simulink library "IO"  (R2025a)
(part 5 of 6)

  raptor_can_rxmsg61 : Raptor_lib/CAN/raptor_can_rxmsg  canDefinition=struct('dbcFile', 'SR26_CAN2.dbc','message', 'BMS_553','comment', '','signals', {{'BMS_counterMsg553','BMS_module5Cell7Volt','BMS_module5Cell8Volt','BMS_module5Cell9Volt'}},'enabled', [ 1 1 1 1;],'scaled', [ 1 1 1 1;],'canBus', '''CAN2''','messageID', [ 553;],'idMask', [ 536870911;],'payloadMask', [],'payloadValue', [],'period', [ 0;],'mailbox', '''''','queueSize', [ 1;],'label', [ 0;],'ver', [ 2;],'showID', [ 0;],'showRaw', [ 0;],'showRawMsg', [ 0;],'useStartVals', [ 0;],'extendedId', [ 0;],'showAge', [ 1;],'useSimFunc', [ 0;],'sim_func_name', '''''','fill', [ 0;],'editID', [ 0;],'signalOrder', [ 2;],'signalAscDes', [ 2;],'msgLength', [ 8;])  canBus='CAN2'  mailbox=''  payloadMask=[]  payloadValue=[]  idMask=hex2dec('1FFFFFFF')  queueSize=1  showID=0  label=0  fill=0  id=553  showRaw=0  showAge=1  signalOrder=2  signalInfo={{struct('Name', 'BMS_module5Cell9Volt','StartBit', [ 48;],'SignalSize', [ 16;],'ByteOrder', 'LittleEndian','ValueType', 'SIGNED','Class', 'int16','Signed', [ 1;],'Factor', [ 0.001;],'Offset', [ 0;],'Min', [ -32.768;],'Max', [ 32.767;],'Units', 'V','StartVal', [ 0;],'Comment', 'Module 5 Cell 9 Voltage','Multiplexed', [ 0;],'Multiplexor', [ 0;],'MultiplexMode_Min', [],'MultiplexMode_Max', []),struct('Name', 'BMS_module5Cell8Volt','StartBit', [ 32;],'SignalSize', [ 16;],'ByteOrder', 'LittleEndian','ValueType', 'SIGNED','Class', 'int16','Signed', [ 1;],'Factor', [ 0.001;],'Offset', [ 0;],'Min', [ -32.768;],'Max', [ 32.767;],'Units', 'V','StartVal', [ 0;],'Comment', 'Module 5 Cell 8 Voltage','Multiplexed', [ 0;],'Multiplexor', [ 0;],'MultiplexMode_Min', [],'MultiplexMode_Max', []),struct('Name', 'BMS_module5Cell7Volt','StartBit', [ 16;],'SignalSize', [ 16;],'ByteOrder', 'LittleEndian','ValueType', 'SIGNED','Class', 'int16','Signed', [ 1;],'Factor', [ 0.001;],'Offset', [ 0;],'Min', [ -32.768;],'Max', [ 32.767;],'Units', 'V','StartVal', [ 0;],'Comment', 'Module 5 Cell 7 Voltage','Multiplexed', [ 0;],'Multiplexor', [ 0;],'MultiplexMode_Min', [],'MultiplexMode_Max', []),struct('Name', 'BMS_counterMsg553','StartBit', [ 0;],'SignalSize', [ 8;],'ByteOrder', 'LittleEndian','ValueType', 'UNSIGNED','Class', 'uint8','Signed', [ 0;],'Factor', [ 1;],'Offset', [ 0;],'Min', [ 0;],'Max', [ 15;],'Units', '','StartVal', [ 0;],'Comment', 'Counter Message 553','Multiplexed', [ 0;],'Multiplexor', [ 0;],'MultiplexMode_Min', [],'MultiplexMode_Max', [])}}  showRawMsg=0  useSimFunc=0  sim_func_name=''  useStartVals=0  extendedId=0
      settings: SourceProductName=Raptor
  raptor_can_rxmsg62 : Raptor_lib/CAN/raptor_can_rxmsg  canDefinition=struct('dbcFile', 'SR26_CAN2.dbc','message', 'BMS_554','comment', '','signals', {{'BMS_counterMsg554','BMS_module5Cell10Volt','BMS_module5Cell11Volt','BMS_module5Cell12Volt'}},'enabled', [ 1 1 1 1;],'scaled', [ 1 1 1 1;],'canBus', '''CAN2''','messageID', [ 554;],'idMask', [ 536870911;],'payloadMask', [],'payloadValue', [],'period', [ 0;],'mailbox', '''''','queueSize', [ 1;],'label', [ 0;],'ver', [ 2;],'showID', [ 0;],'showRaw', [ 0;],'showRawMsg', [ 0;],'useStartVals', [ 0;],'extendedId', [ 0;],'showAge', [ 1;],'useSimFunc', [ 0;],'sim_func_name', '''''','fill', [ 0;],'editID', [ 0;],'signalOrder', [ 2;],'signalAscDes', [ 2;],'msgLength', [ 8;])  canBus='CAN2'  mailbox=''  payloadMask=[]  payloadValue=[]  idMask=hex2dec('1FFFFFFF')  queueSize=1  showID=0  label=0  fill=0  id=554  showRaw=0  showAge=1  signalOrder=2  signalInfo={{struct('Name', 'BMS_module5Cell12Volt','StartBit', [ 48;],'SignalSize', [ 16;],'ByteOrder', 'LittleEndian','ValueType', 'SIGNED','Class', 'int16','Signed', [ 1;],'Factor', [ 0.001;],'Offset', [ 0;],'Min', [ -32.768;],'Max', [ 32.767;],'Units', 'V','StartVal', [ 0;],'Comment', 'Module 5 Cell 12 Voltage','Multiplexed', [ 0;],'Multiplexor', [ 0;],'MultiplexMode_Min', [],'MultiplexMode_Max', []),struct('Name', 'BMS_module5Cell11Volt','StartBit', [ 32;],'SignalSize', [ 16;],'ByteOrder', 'LittleEndian','ValueType', 'SIGNED','Class', 'int16','Signed', [ 1;],'Factor', [ 0.001;],'Offset', [ 0;],'Min', [ -32.768;],'Max', [ 32.767;],'Units', 'V','StartVal', [ 0;],'Comment', 'Module 5 Cell 11 Voltage','Multiplexed', [ 0;],'Multiplexor', [ 0;],'MultiplexMode_Min', [],'MultiplexMode_Max', []),struct('Name', 'BMS_module5Cell10Volt','StartBit', [ 16;],'SignalSize', [ 16;],'ByteOrder', 'LittleEndian','ValueType', 'SIGNED','Class', 'int16','Signed', [ 1;],'Factor', [ 0.001;],'Offset', [ 0;],'Min', [ -32.768;],'Max', [ 32.767;],'Units', 'V','StartVal', [ 0;],'Comment', 'Module 5 Cell 10 Voltage','Multiplexed', [ 0;],'Multiplexor', [ 0;],'MultiplexMode_Min', [],'MultiplexMode_Max', []),struct('Name', 'BMS_counterMsg554','StartBit', [ 0;],'SignalSize', [ 8;],'ByteOrder', 'LittleEndian','ValueType', 'UNSIGNED','Class', 'uint8','Signed', [ 0;],'Factor', [ 1;],'Offset', [ 0;],'Min', [ 0;],'Max', [ 15;],'Units', '','StartVal', [ 0;],'Comment', 'Counter Message 554','Multiplexed', [ 0;],'Multiplexor', [ 0;],'MultiplexMode_Min', [],'MultiplexMode_Max', [])}}  showRawMsg=0  useSimFunc=0  sim_func_name=''  useStartVals=0  extendedId=0
      settings: SourceProductName=Raptor
  raptor_can_rxmsg63 : Raptor_lib/CAN/raptor_can_rxmsg  canDefinition=struct('dbcFile', 'SR26_CAN2.dbc','message', 'BMS_562','comment', '','signals', {{'BMS_counterMsg562','BMS_module5Cell16Temp','BMS_module5Cell17Temp','BMS_module5Cell18Temp'}},'enabled', [ 1 1 1 1;],'scaled', [ 1 1 1 1;],'canBus', '''CAN2''','messageID', [ 562;],'idMask', [ 536870911;],'payloadMask', [],'payloadValue', [],'period', [ 0;],'mailbox', '''''','queueSize', [ 1;],'label', [ 0;],'ver', [ 2;],'showID', [ 0;],'showRaw', [ 0;],'showRawMsg', [ 0;],'useStartVals', [ 0;],'extendedId', [ 0;],'showAge', [ 1;],'useSimFunc', [ 0;],'sim_func_name', '''''','fill', [ 0;],'editID', [ 0;],'signalOrder', [ 1;],'signalAscDes', [ 1;],'msgLength', [ 8;])  canBus='CAN2'  mailbox=''  payloadMask=[]  payloadValue=[]  idMask=hex2dec('1FFFFFFF')  queueSize=1  showID=0  label=0  fill=0  id=562  showRaw=0  showAge=1  signalOrder=1  signalInfo={{struct('Name', 'BMS_module5Cell18Temp','StartBit', [ 48;],'SignalSize', [ 16;],'ByteOrder', 'LittleEndian','ValueType', 'SIGNED','Class', 'int16','Signed', [ 1;],'Factor', [ 0.1;],'Offset', [ 0;],'Min', [ -3276.8;],'Max', [ 3276.7;],'Units', 'degC','StartVal', [ 0;],'Comment', 'Module 5 Cell 18 Temperature','Multiplexed', [ 0;],'Multiplexor', [ 0;],'MultiplexMode_Min', [],'MultiplexMode_Max', []),struct('Name', 'BMS_module5Cell17Temp','StartBit', [ 32;],'SignalSize', [ 16;],'ByteOrder', 'LittleEndian','ValueType', 'SIGNED','Class', 'int16','Signed', [ 1;],'Factor', [ 0.1;],'Offset', [ 0;],'Min', [ -3276.8;],'Max', [ 3276.7;],'Units', 'degC','StartVal', [ 0;],'Comment', 'Module 5 Cell 17 Temperature','Multiplexed', [ 0;],'Multiplexor', [ 0;],'MultiplexMode_Min', [],'MultiplexMode_Max', []),struct('Name', 'BMS_module5Cell16Temp','StartBit', [ 16;],'SignalSize', [ 16;],'ByteOrder', 'LittleEndian','ValueType', 'SIGNED','Class', 'int16','Signed', [ 1;],'Factor', [ 0.1;],'Offset', [ 0;],'Min', [ -3276.8;],'Max', [ 3276.7;],'Units', 'degC','StartVal', [ 0;],'Comment', 'Module 5 Cell 16 Temperature','Multiplexed', [ 0;],'Multiplexor', [ 0;],'MultiplexMode_Min', [],'MultiplexMode_Max', []),struct('Name', 'BMS_counterMsg562','StartBit', [ 0;],'SignalSize', [ 8;],'ByteOrder', 'LittleEndian','ValueType', 'UNSIGNED','Class', 'uint8','Signed', [ 0;],'Factor', [ 1;],'Offset', [ 0;],'Min', [ 0;],'Max', [ 15;],'Units', '','StartVal', [ 0;],'Comment', 'Counter Message 562','Multiplexed', [ 0;],'Multiplexor', [ 0;],'MultiplexMode_Min', [],'MultiplexMode_Max', [])}}  showRawMsg=0  useSimFunc=0  sim_func_name=''  useStartVals=0  extendedId=0
      settings: SourceProductName=Raptor
  raptor_can_rxmsg64 : Raptor_lib/CAN/raptor_can_rxmsg  canDefinition=struct('dbcFile', 'SR26_CAN2.dbc','message', 'BMS_561','comment', '','signals', {{'BMS_counterMsg561','BMS_module5Cell13Temp','BMS_module5Cell14Temp','BMS_module5Cell15Temp'}},'enabled', [ 1 1 1 1;],'scaled', [ 1 1 1 1;],'canBus', '''CAN2''','messageID', [ 561;],'idMask', [ 536870911;],'payloadMask', [],'payloadValue', [],'period', [ 0;],'mailbox', '''''','queueSize', [ 1;],'label', [ 0;],'ver', [ 2;],'showID', [ 0;],'showRaw', [ 0;],'showRawMsg', [ 0;],'useStartVals', [ 0;],'extendedId', [ 0;],'showAge', [ 1;],'useSimFunc', [ 0;],'sim_func_name', '''''','fill', [ 0;],'editID', [ 0;],'signalOrder', [ 1;],'signalAscDes', [ 1;],'msgLength', [ 8;])  canBus='CAN2'  mailbox=''  payloadMask=[]  payloadValue=[]  idMask=hex2dec('1FFFFFFF')  queueSize=1  showID=0  label=0  fill=0  id=561  showRaw=0  showAge=1  signalOrder=1  signalInfo={{struct('Name', 'BMS_module5Cell15Temp','StartBit', [ 48;],'SignalSize', [ 16;],'ByteOrder', 'LittleEndian','ValueType', 'SIGNED','Class', 'int16','Signed', [ 1;],'Factor', [ 0.1;],'Offset', [ 0;],'Min', [ -3276.8;],'Max', [ 3276.7;],'Units', 'degC','StartVal', [ 0;],'Comment', 'Module 5 Cell 15 Temperature','Multiplexed', [ 0;],'Multiplexor', [ 0;],'MultiplexMode_Min', [],'MultiplexMode_Max', []),struct('Name', 'BMS_module5Cell14Temp','StartBit', [ 32;],'SignalSize', [ 16;],'ByteOrder', 'LittleEndian','ValueType', 'SIGNED','Class', 'int16','Signed', [ 1;],'Factor', [ 0.1;],'Offset', [ 0;],'Min', [ -3276.8;],'Max', [ 3276.7;],'Units', 'degC','StartVal', [ 0;],'Comment', 'Module 5 Cell 14 Temperature','Multiplexed', [ 0;],'Multiplexor', [ 0;],'MultiplexMode_Min', [],'MultiplexMode_Max', []),struct('Name', 'BMS_module5Cell13Temp','StartBit', [ 16;],'SignalSize', [ 16;],'ByteOrder', 'LittleEndian','ValueType', 'SIGNED','Class', 'int16','Signed', [ 1;],'Factor', [ 0.1;],'Offset', [ 0;],'Min', [ -3276.8;],'Max', [ 3276.7;],'Units', 'degC','StartVal', [ 0;],'Comment', 'Module 5 Cell 13 Temperature','Multiplexed', [ 0;],'Multiplexor', [ 0;],'MultiplexMode_Min', [],'MultiplexMode_Max', []),struct('Name', 'BMS_counterMsg561','StartBit', [ 0;],'SignalSize', [ 8;],'ByteOrder', 'LittleEndian','ValueType', 'UNSIGNED','Class', 'uint8','Signed', [ 0;],'Factor', [ 1;],'Offset', [ 0;],'Min', [ 0;],'Max', [ 15;],'Units', '','StartVal', [ 0;],'Comment', 'Counter Message 561','Multiplexed', [ 0;],'Multiplexor', [ 0;],'MultiplexMode_Min', [],'MultiplexMode_Max', [])}}  showRawMsg=0  useSimFunc=0  sim_func_name=''  useStartVals=0  extendedId=0
      settings: SourceProductName=Raptor
  raptor_can_rxmsg65 : Raptor_lib/CAN/raptor_can_rxmsg  canDefinition=struct('dbcFile', 'SR26_CAN2.dbc','message', 'BMS_506','comment', '','signals', {{'BMS_counterMsg506','BMS_module1Cell10Volt','BMS_module1Cell11Volt','BMS_module1Cell12Volt'}},'enabled', [ 1 1 1 1;],'scaled', [ 1 1 1 1;],'canBus', '''CAN2''','messageID', [ 506;],'idMask', [ 536870911;],'payloadMask', [],'payloadValue', [],'period', [ 0;],'mailbox', '''''','queueSize', [ 1;],'label', [ 0;],'ver', [ 2;],'showID', [ 0;],'showRaw', [ 0;],'showRawMsg', [ 0;],'useStartVals', [ 0;],'extendedId', [ 0;],'showAge', [ 1;],'useSimFunc', [ 0;],'sim_func_name', '''''','fill', [ 0;],'editID', [ 0;],'signalOrder', [ 2;],'signalAscDes', [ 2;],'msgLength', [ 8;])  canBus='CAN2'  mailbox=''  payloadMask=[]  payloadValue=[]  idMask=hex2dec('1FFFFFFF')  queueSize=1  showID=0  label=0  fill=0  id=506  showRaw=0  showAge=1  signalOrder=2  signalInfo={{struct('Name', 'BMS_module1Cell12Volt','StartBit', [ 48;],'SignalSize', [ 16;],'ByteOrder', 'LittleEndian','ValueType', 'SIGNED','Class', 'int16','Signed', [ 1;],'Factor', [ 0.001;],'Offset', [ 0;],'Min', [ -32.768;],'Max', [ 32.767;],'Units', 'V','StartVal', [ 0;],'Comment', 'Module 1 Cell 12 Voltage','Multiplexed', [ 0;],'Multiplexor', [ 0;],'MultiplexMode_Min', [],'MultiplexMode_Max', []),struct('Name', 'BMS_module1Cell11Volt','StartBit', [ 32;],'SignalSize', [ 16;],'ByteOrder', 'LittleEndian','ValueType', 'SIGNED','Class', 'int16','Signed', [ 1;],'Factor', [ 0.001;],'Offset', [ 0;],'Min', [ -32.768;],'Max', [ 32.767;],'Units', 'V','StartVal', [ 0;],'Comment', 'Module 1 Cell 11 Voltage','Multiplexed', [ 0;],'Multiplexor', [ 0;],'MultiplexMode_Min', [],'MultiplexMode_Max', []),struct('Name', 'BMS_module1Cell10Volt','StartBit', [ 16;],'SignalSize', [ 16;],'ByteOrder', 'LittleEndian','ValueType', 'SIGNED','Class', 'int16','Signed', [ 1;],'Factor', [ 0.001;],'Offset', [ 0;],'Min', [ -32.768;],'Max', [ 32.767;],'Units', 'V','StartVal', [ 0;],'Comment', 'Module 1 Cell 10 Voltage','Multiplexed', [ 0;],'Multiplexor', [ 0;],'MultiplexMode_Min', [],'MultiplexMode_Max', []),struct('Name', 'BMS_counterMsg506','StartBit', [ 0;],'SignalSize', [ 8;],'ByteOrder', 'LittleEndian','ValueType', 'UNSIGNED','Class', 'uint8','Signed', [ 0;],'Factor', [ 1;],'Offset', [ 0;],'Min', [ 0;],'Max', [ 15;],'Units', '','StartVal', [ 0;],'Comment', 'Counter Message 506','Multiplexed', [ 0;],'Multiplexor', [ 0;],'MultiplexMode_Min', [],'MultiplexMode_Max', [])}}  showRawMsg=0  useSimFunc=0  sim_func_name=''  useStartVals=0  extendedId=0
      settings: SourceProductName=Raptor
  raptor_can_rxmsg66 : Raptor_lib/CAN/raptor_can_rxmsg  canDefinition=struct('dbcFile', 'SR26_CAN2.dbc','message', 'BMS_507','comment', '','signals', {{'BMS_counterMsg507','BMS_module1Cell13Volt','BMS_module1Cell14Volt','BMS_module1Cell15Volt'}},'enabled', [ 1 1 1 1;],'scaled', [ 1 1 1 1;],'canBus', '''CAN2''','messageID', [ 507;],'idMask', [ 536870911;],'payloadMask', [],'payloadValue', [],'period', [ 0;],'mailbox', '''''','queueSize', [ 1;],'label', [ 0;],'ver', [ 2;],'showID', [ 0;],'showRaw', [ 0;],'showRawMsg', [ 0;],'useStartVals', [ 0;],'extendedId', [ 0;],'showAge', [ 1;],'useSimFunc', [ 0;],'sim_func_name', '''''','fill', [ 0;],'editID', [ 0;],'signalOrder', [ 2;],'signalAscDes', [ 2;],'msgLength', [ 8;])  canBus='CAN2'  mailbox=''  payloadMask=[]  payloadValue=[]  idMask=hex2dec('1FFFFFFF')  queueSize=1  showID=0  label=0  fill=0  id=507  showRaw=0  showAge=1  signalOrder=2  signalInfo={{struct('Name', 'BMS_module1Cell15Volt','StartBit', [ 48;],'SignalSize', [ 16;],'ByteOrder', 'LittleEndian','ValueType', 'SIGNED','Class', 'int16','Signed', [ 1;],'Factor', [ 0.001;],'Offset', [ 0;],'Min', [ -32.768;],'Max', [ 32.767;],'Units', 'V','StartVal', [ 0;],'Comment', 'Module 1 Cell 15 Voltage','Multiplexed', [ 0;],'Multiplexor', [ 0;],'MultiplexMode_Min', [],'MultiplexMode_Max', []),struct('Name', 'BMS_module1Cell14Volt','StartBit', [ 32;],'SignalSize', [ 16;],'ByteOrder', 'LittleEndian','ValueType', 'SIGNED','Class', 'int16','Signed', [ 1;],'Factor', [ 0.001;],'Offset', [ 0;],'Min', [ -32.768;],'Max', [ 32.767;],'Units', 'V','StartVal', [ 0;],'Comment', 'Module 1 Cell 14 Voltage','Multiplexed', [ 0;],'Multiplexor', [ 0;],'MultiplexMode_Min', [],'MultiplexMode_Max', []),struct('Name', 'BMS_module1Cell13Volt','StartBit', [ 16;],'SignalSize', [ 16;],'ByteOrder', 'LittleEndian','ValueType', 'SIGNED','Class', 'int16','Signed', [ 1;],'Factor', [ 0.001;],'Offset', [ 0;],'Min', [ -32.768;],'Max', [ 32.767;],'Units', 'V','StartVal', [ 0;],'Comment', 'Module 1 Cell 13 Voltage','Multiplexed', [ 0;],'Multiplexor', [ 0;],'MultiplexMode_Min', [],'MultiplexMode_Max', []),struct('Name', 'BMS_counterMsg507','StartBit', [ 0;],'SignalSize', [ 8;],'ByteOrder', 'LittleEndian','ValueType', 'UNSIGNED','Class', 'uint8','Signed', [ 0;],'Factor', [ 1;],'Offset', [ 0;],'Min', [ 0;],'Max', [ 15;],'Units', '','StartVal', [ 0;],'Comment', 'Counter Message 507','Multiplexed', [ 0;],'Multiplexor', [ 0;],'MultiplexMode_Min', [],'MultiplexMode_Max', [])}}  showRawMsg=0  useSimFunc=0  sim_func_name=''  useStartVals=0  extendedId=0
      settings: SourceProductName=Raptor
  raptor_can_rxmsg67 : Raptor_lib/CAN/raptor_can_rxmsg  canDefinition=struct('dbcFile', 'SR26_CAN2.dbc','message', 'BMS_508','comment', '','signals', {{'BMS_counterMsg508','BMS_module1Cell16Volt','BMS_module1Cell17Volt','BMS_module1Cell18Volt'}},'enabled', [ 1 1 1 1;],'scaled', [ 1 1 1 1;],'canBus', '''CAN2''','messageID', [ 508;],'idMask', [ 536870911;],'payloadMask', [],'payloadValue', [],'period', [ 0;],'mailbox', '''''','queueSize', [ 1;],'label', [ 0;],'ver', [ 2;],'showID', [ 0;],'showRaw', [ 0;],'showRawMsg', [ 0;],'useStartVals', [ 0;],'extendedId', [ 0;],'showAge', [ 1;],'useSimFunc', [ 0;],'sim_func_name', '''''','fill', [ 0;],'editID', [ 0;],'signalOrder', [ 2;],'signalAscDes', [ 2;],'msgLength', [ 8;])  canBus='CAN2'  mailbox=''  payloadMask=[]  payloadValue=[]  idMask=hex2dec('1FFFFFFF')  queueSize=1  showID=0  label=0  fill=0  id=508  showRaw=0  showAge=1  signalOrder=2  signalInfo={{struct('Name', 'BMS_module1Cell18Volt','StartBit', [ 48;],'SignalSize', [ 16;],'ByteOrder', 'LittleEndian','ValueType', 'SIGNED','Class', 'int16','Signed', [ 1;],'Factor', [ 0.001;],'Offset', [ 0;],'Min', [ -32.768;],'Max', [ 32.767;],'Units', 'V','StartVal', [ 0;],'Comment', 'Module 1 Cell 18 Voltage','Multiplexed', [ 0;],'Multiplexor', [ 0;],'MultiplexMode_Min', [],'MultiplexMode_Max', []),struct('Name', 'BMS_module1Cell17Volt','StartBit', [ 32;],'SignalSize', [ 16;],'ByteOrder', 'LittleEndian','ValueType', 'SIGNED','Class', 'int16','Signed', [ 1;],'Factor', [ 0.001;],'Offset', [ 0;],'Min', [ -32.768;],'Max', [ 32.767;],'Units', 'V','StartVal', [ 0;],'Comment', 'Module 1 Cell 17 Voltage','Multiplexed', [ 0;],'Multiplexor', [ 0;],'MultiplexMode_Min', [],'MultiplexMode_Max', []),struct('Name', 'BMS_module1Cell16Volt','StartBit', [ 16;],'SignalSize', [ 16;],'ByteOrder', 'LittleEndian','ValueType', 'SIGNED','Class', 'int16','Signed', [ 1;],'Factor', [ 0.001;],'Offset', [ 0;],'Min', [ -32.768;],'Max', [ 32.767;],'Units', 'V','StartVal', [ 0;],'Comment', 'Module 1 Cell 16 Voltage','Multiplexed', [ 0;],'Multiplexor', [ 0;],'MultiplexMode_Min', [],'MultiplexMode_Max', []),struct('Name', 'BMS_counterMsg508','StartBit', [ 0;],'SignalSize', [ 8;],'ByteOrder', 'LittleEndian','ValueType', 'UNSIGNED','Class', 'uint8','Signed', [ 0;],'Factor', [ 1;],'Offset', [ 0;],'Min', [ 0;],'Max', [ 15;],'Units', '','StartVal', [ 0;],'Comment', 'Counter Message 508','Multiplexed', [ 0;],'Multiplexor', [ 0;],'MultiplexMode_Min', [],'MultiplexMode_Max', [])}}  showRawMsg=0  useSimFunc=0  sim_func_name=''  useStartVals=0  extendedId=0
      settings: SourceProductName=Raptor
  raptor_can_rxmsg7 : Raptor_lib/CAN/raptor_can_rxmsg  canDefinition=struct('dbcFile', 'SR26_CAN2.dbc','message', 'BMS_502','comment', '','signals', {{'BMS_counterMsg502','BMS_module4Volt','BMS_module5Volt'}},'enabled', [ 1 1 1;],'scaled', [ 1 1 1;],'canBus', '''CAN2''','messageID', [ 502;],'idMask', [ 536870911;],'payloadMask', [],'payloadValue', [],'period', [ 0;],'mailbox', '''''','queueSize', [ 1;],'label', [ 0;],'ver', [ 2;],'showID', [ 0;],'showRaw', [ 0;],'showRawMsg', [ 0;],'useStartVals', [ 0;],'extendedId', [ 0;],'showAge', [ 1;],'useSimFunc', [ 0;],'sim_func_name', '''''','fill', [ 0;],'editID', [ 0;],'signalOrder', [ 2;],'signalAscDes', [ 2;],'msgLength', [ 8;])  canBus='CAN2'  mailbox=''  payloadMask=[]  payloadValue=[]  idMask=hex2dec('1FFFFFFF')  queueSize=1  showID=0  label=0  fill=0  id=502  showRaw=0  showAge=1  signalOrder=2  signalInfo={{struct('Name', 'BMS_module5Volt','StartBit', [ 32;],'SignalSize', [ 16;],'ByteOrder', 'LittleEndian','ValueType', 'SIGNED','Class', 'int16','Signed', [ 1;],'Factor', [ 0.001;],'Offset', [ 0;],'Min', [ -32.768;],'Max', [ 32.767;],'Units', 'V','StartVal', [ 0;],'Comment', 'Module 5 Voltage','Multiplexed', [ 0;],'Multiplexor', [ 0;],'MultiplexMode_Min', [],'MultiplexMode_Max', []),struct('Name', 'BMS_module4Volt','StartBit', [ 16;],'SignalSize', [ 16;],'ByteOrder', 'LittleEndian','ValueType', 'SIGNED','Class', 'int16','Signed', [ 1;],'Factor', [ 0.001;],'Offset', [ 0;],'Min', [ -32.768;],'Max', [ 32.767;],'Units', 'V','StartVal', [ 0;],'Comment', 'Module 4 Voltage','Multiplexed', [ 0;],'Multiplexor', [ 0;],'MultiplexMode_Min', [],'MultiplexMode_Max', []),struct('Name', 'BMS_counterMsg502','StartBit', [ 0;],'SignalSize', [ 8;],'ByteOrder', 'LittleEndian','ValueType', 'UNSIGNED','Class', 'uint8','Signed', [ 0;],'Factor', [ 1;],'Offset', [ 0;],'Min', [ 0;],'Max', [ 15;],'Units', '','StartVal', [ 0;],'Comment', 'Counter Message 502','Multiplexed', [ 0;],'Multiplexor', [ 0;],'MultiplexMode_Min', [],'MultiplexMode_Max', [])}}  showRawMsg=0  useSimFunc=0  sim_func_name=''  useStartVals=0  extendedId=0
      settings: SourceProductName=Raptor
  raptor_can_rxmsg8 : Raptor_lib/CAN/raptor_can_rxmsg  canDefinition=struct('dbcFile', 'SR26_CAN2.dbc','message', 'BMS_503','comment', '','signals', {{'BMS_counterMsg503','BMS_module1Cell1Volt','BMS_module1Cell2Volt','BMS_module1Cell3Volt'}},'enabled', [ 1 1 1 1;],'scaled', [ 1 1 1 1;],'canBus', '''CAN2''','messageID', [ 503;],'idMask', [ 536870911;],'payloadMask', [],'payloadValue', [],'period', [ 0;],'mailbox', '''''','queueSize', [ 1;],'label', [ 0;],'ver', [ 2;],'showID', [ 0;],'showRaw', [ 0;],'showRawMsg', [ 0;],'useStartVals', [ 0;],'extendedId', [ 0;],'showAge', [ 1;],'useSimFunc', [ 0;],'sim_func_name', '''''','fill', [ 0;],'editID', [ 0;],'signalOrder', [ 2;],'signalAscDes', [ 2;],'msgLength', [ 8;])  canBus='CAN2'  mailbox=''  payloadMask=[]  payloadValue=[]  idMask=hex2dec('1FFFFFFF')  queueSize=1  showID=0  label=0  fill=0  id=503  showRaw=0  showAge=1  signalOrder=2  signalInfo={{struct('Name', 'BMS_module1Cell3Volt','StartBit', [ 48;],'SignalSize', [ 16;],'ByteOrder', 'LittleEndian','ValueType', 'SIGNED','Class', 'int16','Signed', [ 1;],'Factor', [ 0.001;],'Offset', [ 0;],'Min', [ -32.768;],'Max', [ 32.767;],'Units', 'V','StartVal', [ 0;],'Comment', 'Module 1 Cell 3 Voltage','Multiplexed', [ 0;],'Multiplexor', [ 0;],'MultiplexMode_Min', [],'MultiplexMode_Max', []),struct('Name', 'BMS_module1Cell2Volt','StartBit', [ 32;],'SignalSize', [ 16;],'ByteOrder', 'LittleEndian','ValueType', 'SIGNED','Class', 'int16','Signed', [ 1;],'Factor', [ 0.001;],'Offset', [ 0;],'Min', [ -32.768;],'Max', [ 32.767;],'Units', 'V','StartVal', [ 0;],'Comment', 'Module 1 Cell 2 Voltage','Multiplexed', [ 0;],'Multiplexor', [ 0;],'MultiplexMode_Min', [],'MultiplexMode_Max', []),struct('Name', 'BMS_module1Cell1Volt','StartBit', [ 16;],'SignalSize', [ 16;],'ByteOrder', 'LittleEndian','ValueType', 'SIGNED','Class', 'int16','Signed', [ 1;],'Factor', [ 0.001;],'Offset', [ 0;],'Min', [ -32.768;],'Max', [ 32.767;],'Units', 'V','StartVal', [ 0;],'Comment', 'Module 1 Cell 1 Voltage','Multiplexed', [ 0;],'Multiplexor', [ 0;],'MultiplexMode_Min', [],'MultiplexMode_Max', []),struct('Name', 'BMS_counterMsg503','StartBit', [ 0;],'SignalSize', [ 8;],'ByteOrder', 'LittleEndian','ValueType', 'UNSIGNED','Class', 'uint8','Signed', [ 0;],'Factor', [ 1;],'Offset', [ 0;],'Min', [ 0;],'Max', [ 15;],'Units', '','StartVal', [ 0;],'Comment', 'Counter Message 503','Multiplexed', [ 0;],'Multiplexor', [ 0;],'MultiplexMode_Min', [],'MultiplexMode_Max', [])}}  showRawMsg=0  useSimFunc=0  sim_func_name=''  useStartVals=0  extendedId=0
      settings: SourceProductName=Raptor
  raptor_can_rxmsg9 : Raptor_lib/CAN/raptor_can_rxmsg  canDefinition=struct('dbcFile', 'SR26_CAN2.dbc','message', 'BMS_504','comment', '','signals', {{'BMS_counterMsg504','BMS_module1Cell4Volt','BMS_module1Cell5Volt','BMS_module1Cell6Volt'}},'enabled', [ 1 1 1 1;],'scaled', [ 1 1 1 1;],'canBus', '''CAN2''','messageID', [ 504;],'idMask', [ 536870911;],'payloadMask', [],'payloadValue', [],'period', [ 0;],'mailbox', '''''','queueSize', [ 1;],'label', [ 0;],'ver', [ 2;],'showID', [ 0;],'showRaw', [ 0;],'showRawMsg', [ 0;],'useStartVals', [ 0;],'extendedId', [ 0;],'showAge', [ 1;],'useSimFunc', [ 0;],'sim_func_name', '''''','fill', [ 0;],'editID', [ 0;],'signalOrder', [ 2;],'signalAscDes', [ 2;],'msgLength', [ 8;])  canBus='CAN2'  mailbox=''  payloadMask=[]  payloadValue=[]  idMask=hex2dec('1FFFFFFF')  queueSize=1  showID=0  label=0  fill=0  id=504  showRaw=0  showAge=1  signalOrder=2  signalInfo={{struct('Name', 'BMS_module1Cell6Volt','StartBit', [ 48;],'SignalSize', [ 16;],'ByteOrder', 'LittleEndian','ValueType', 'SIGNED','Class', 'int16','Signed', [ 1;],'Factor', [ 0.001;],'Offset', [ 0;],'Min', [ -32.768;],'Max', [ 32.767;],'Units', 'V','StartVal', [ 0;],'Comment', 'Module 1 Cell 6 Voltage','Multiplexed', [ 0;],'Multiplexor', [ 0;],'MultiplexMode_Min', [],'MultiplexMode_Max', []),struct('Name', 'BMS_module1Cell5Volt','StartBit', [ 32;],'SignalSize', [ 16;],'ByteOrder', 'LittleEndian','ValueType', 'SIGNED','Class', 'int16','Signed', [ 1;],'Factor', [ 0.001;],'Offset', [ 0;],'Min', [ -32.768;],'Max', [ 32.767;],'Units', 'V','StartVal', [ 0;],'Comment', 'Module 1 Cell 5 Voltage','Multiplexed', [ 0;],'Multiplexor', [ 0;],'MultiplexMode_Min', [],'MultiplexMode_Max', []),struct('Name', 'BMS_module1Cell4Volt','StartBit', [ 16;],'SignalSize', [ 16;],'ByteOrder', 'LittleEndian','ValueType', 'SIGNED','Class', 'int16','Signed', [ 1;],'Factor', [ 0.001;],'Offset', [ 0;],'Min', [ -32.768;],'Max', [ 32.767;],'Units', 'V','StartVal', [ 0;],'Comment', 'Module 1 Cell 4 Voltage','Multiplexed', [ 0;],'Multiplexor', [ 0;],'MultiplexMode_Min', [],'MultiplexMode_Max', []),struct('Name', 'BMS_counterMsg504','StartBit', [ 0;],'SignalSize', [ 8;],'ByteOrder', 'LittleEndian','ValueType', 'UNSIGNED','Class', 'uint8','Signed', [ 0;],'Factor', [ 1;],'Offset', [ 0;],'Min', [ 0;],'Max', [ 15;],'Units', '','StartVal', [ 0;],'Comment', 'Counter Message 504','Multiplexed', [ 0;],'Multiplexor', [ 0;],'MultiplexMode_Min', [],'MultiplexMode_Max', [])}}  showRawMsg=0  useSimFunc=0  sim_func_name=''  useStartVals=0  extendedId=0
      settings: SourceProductName=Raptor
  IO_CAN2_BMS_Bus : Outport
  wires:
  Bus Creator36/1 -> Bus Creator5/45  "IO_CAN2_544_Bus"
  Bus Creator47/1 -> Bus Creator5/44  "IO_CAN2_543_Bus"
  raptor_can_rxmsg56/1 -> Bus Creator57/1  "Age"
  raptor_can_rxmsg23/5 -> Bus Creator23/5  "BMS_module2Cell15Temp"
  raptor_can_rxmsg24/1 -> Bus Creator24/1  "Age"
  raptor_can_rxmsg19/2 -> Bus Creator19/2  "BMS_counterMsg521"
  raptor_can_rxmsg48/2 -> Bus Creator48/2  "BMS_counterMsg527"
  raptor_can_rxmsg40/1 -> Bus Creator40/1  "Age"
  raptor_can_rxmsg28/4 -> Bus Creator28/4  "BMS_module5Cell14Volt"
  raptor_can_rxmsg57/4 -> Bus Creator58/4  "BMS_module4Cell17Temp"
  raptor_can_rxmsg14/5 -> Bus Creator14/5  "BMS_module1Cell12Temp"
  raptor_can_rxmsg43/5 -> Bus Creator43/5  "BMS_module4Cell3Volt"
  Bus Creator10/1 -> Bus Creator5/10  "IO_CAN2_509_Bus"
  raptor_can_rxmsg48/3 -> Bus Creator48/3  "BMS_module3Cell1Volt"
  raptor_can_rxmsg63/3 -> Bus Creator64/3  "BMS_module5Cell16Temp"
  raptor_can_rxmsg63/2 -> Bus Creator64/2  "BMS_counterMsg562"
  raptor_can_rxmsg30/2 -> Bus Creator30/2  "BMS_counterMsg538"
  Bus Creator37/1 -> Bus Creator5/50  "IO_CAN2_549_Bus"
  raptor_can_rxmsg43/4 -> Bus Creator43/4  "BMS_module4Cell2Volt"
  raptor_can_rxmsg33/2 -> Bus Creator33/2  "BMS_counterMsg535"
  raptor_can_rxmsg14/3 -> Bus Creator14/3  "BMS_module1Cell10Temp"
  raptor_can_rxmsg64/1 -> Bus Creator65/1  "Age"
  raptor_can_rxmsg59/5 -> Bus Creator60/5  "BMS_module5Cell6Volt"
  raptor_can_rxmsg25/3 -> Bus Creator25/3  "BMS_module2Cell7Volt"
  raptor_can_rxmsg62/5 -> Bus Creator63/5  "BMS_module5Cell12Volt"
  raptor_can_rxmsg10/4 -> Bus Creator10/4  "BMS_module1Cell2Temp"
  raptor_can_rxmsg33/3 -> Bus Creator33/3  "BMS_module3Cell7Temp"
  raptor_can_rxmsg35/3 -> Bus Creator35/3  "BMS_module3Cell13Temp"
  raptor_can_rxmsg64/2 -> Bus Creator65/2  "BMS_counterMsg561"
  raptor_can_rxmsg52/2 -> Bus Creator53/2  "BMS_counterMsg531"
  raptor_can_rxmsg5/5 -> Bus Creator6/5  "BMS_packSOC"
  raptor_can_rxmsg16/4 -> Bus Creator16/4  "BMS_module1Cell17Temp"
  raptor_can_rxmsg19/4 -> Bus Creator19/4  "BMS_module2Cell2Temp"
  raptor_can_rxmsg7/4 -> Bus Creator8/4  "BMS_module5Volt"
  Bus Creator24/1 -> Bus Creator5/17  "IO_CAN2_516_Bus"
  raptor_can_rxmsg42/1 -> Bus Creator42/1  "Age"
  raptor_can_rxmsg35/1 -> Bus Creator35/1  "Age"
  Bus Creator5/1 -> IO_CAN2_BMS_Bus/1  "IO_CAN2_BMS_Bus"
  Bus Creator68/1 -> Bus Creator5/9  "IO_CAN2_508_Bus"
  Bus Creator51/1 -> Bus Creator5/30  "IO_CAN2_529_Bus"
  raptor_can_rxmsg55/1 -> Bus Creator56/1  "Age"
  Bus Creator14/1 -> Bus Creator5/13  "IO_CAN2_512_Bus"
  raptor_can_rxmsg47/4 -> Bus Creator47/4  "BMS_module4Cell14Volt"
  raptor_can_rxmsg58/3 -> Bus Creator59/3  "BMS_module5Cell1Volt"
  raptor_can_rxmsg23/1 -> Bus Creator23/1  "Age"
  raptor_can_rxmsg38/5 -> Bus Creator38/5  "BMS_module4Cell3Temp"
  raptor_can_rxmsg43/2 -> Bus Creator43/2  "BMS_counterMsg539"
  raptor_can_rxmsg27/5 -> Bus Creator27/5  "BMS_module2Cell15Volt"
  Bus Creator44/1 -> Bus Creator5/41  "IO_CAN2_540_Bus"
  raptor_can_rxmsg55/4 -> Bus Creator56/4  "BMS_module5Cell5Temp"
  raptor_can_rxmsg44/5 -> Bus Creator44/5  "BMS_module4Cell6Volt"
  raptor_can_rxmsg20/2 -> Bus Creator20/2  "BMS_counterMsg522"
  raptor_can_rxmsg35/2 -> Bus Creator35/2  "BMS_counterMsg537"
  Bus Creator66/1 -> Bus Creator5/7  "IO_CAN2_506_Bus"
  raptor_can_rxmsg22/1 -> Bus Creator22/1  "Age"
  raptor_can_rxmsg59/4 -> Bus Creator60/4  "BMS_module5Cell5Volt"
  raptor_can_rxmsg14/1 -> Bus Creator14/1  "Age"
  raptor_can_rxmsg8/3 -> Bus Creator9/3  "BMS_module1Cell1Volt"
  raptor_can_rxmsg37/1 -> Bus Creator37/1  "Age"
  raptor_can_rxmsg11/1 -> Bus Creator11/1  "Age"
  raptor_can_rxmsg26/4 -> Bus Creator26/4  "BMS_module2Cell11Volt"
  raptor_can_rxmsg59/2 -> Bus Creator60/2  "BMS_counterMsg552"
  raptor_can_rxmsg64/3 -> Bus Creator65/3  "BMS_module5Cell13Temp"
  raptor_can_rxmsg39/5 -> Bus Creator39/5  "BMS_module5Cell12Temp"
  raptor_can_rxmsg16/1 -> Bus Creator16/1  "Age"
  raptor_can_rxmsg57/2 -> Bus Creator58/2  "BMS_counterMsg550"
  raptor_can_rxmsg24/2 -> Bus Creator24/2  "BMS_counterMsg516"
  raptor_can_rxmsg6/2 -> Bus Creator7/2  "BMS_counterMsg501"
  raptor_can_rxmsg24/4 -> Bus Creator24/4  "BMS_module2Cell5Volt"
  Bus Creator48/1 -> Bus Creator5/28  "IO_CAN2_527_Bus"
  raptor_can_rxmsg6/4 -> Bus Creator7/4  "BMS_module2Volt"
  raptor_can_rxmsg59/3 -> Bus Creator60/3  "BMS_module5Cell4Volt"
  raptor_can_rxmsg60/5 -> Bus Creator61/5  "BMS_module1Cell9Volt"
  raptor_can_rxmsg6/5 -> Bus Creator7/5  "BMS_module3Volt"
  raptor_can_rxmsg15/1 -> Bus Creator15/1  "Age"
  raptor_can_rxmsg17/5 -> Bus Creator17/5  "BMS_module2Cell18Volt"
  raptor_can_rxmsg29/1 -> Bus Creator29/1  "Age"
  raptor_can_rxmsg10/2 -> Bus Creator10/2  "BMS_counterMsg509"
  Bus Creator17/1 -> Bus Creator5/21  "IO_CAN2_520_Bus"
  raptor_can_rxmsg17/1 -> Bus Creator17/1  "Age"
  raptor_can_rxmsg27/3 -> Bus Creator27/3  "BMS_module2Cell13Volt"
  raptor_can_rxmsg49/5 -> Bus Creator49/5  "BMS_module3Cell6Volt"
  raptor_can_rxmsg40/5 -> Bus Creator40/5  "BMS_module4Cell6Temp"
  raptor_can_rxmsg26/5 -> Bus Creator26/5  "BMS_module2Cell12Volt"
  raptor_can_rxmsg38/3 -> Bus Creator38/3  "BMS_module4Cell1Temp"
  Bus Creator39/1 -> Bus Creator5/61  "IO_CAN2_560_Bus"
  raptor_can_rxmsg16/5 -> Bus Creator16/5  "BMS_module1Cell18Temp"
  raptor_can_rxmsg48/4 -> Bus Creator48/4  "BMS_module3Cell2Volt"
  Bus Creator13/1 -> Bus Creator5/12  "IO_CAN2_511_Bus"
  raptor_can_rxmsg66/1 -> Bus Creator67/1  "Age"
  raptor_can_rxmsg63/4 -> Bus Creator64/4  "BMS_module5Cell17Temp"
  raptor_can_rxmsg53/2 -> Bus Creator54/2  "BMS_counterMsg556"
  raptor_can_rxmsg51/5 -> Bus Creator52/5  "BMS_module3Cell12Volt"
  raptor_can_rxmsg18/4 -> Bus Creator18/4  "BMS_module2Cell17Temp"
  raptor_can_rxmsg46/1 -> Bus Creator46/1  "Age"
  raptor_can_rxmsg67/1 -> Bus Creator68/1  "Age"
  raptor_can_rxmsg57/5 -> Bus Creator58/5  "BMS_module4Cell18Temp"
  raptor_can_rxmsg36/1 -> Bus Creator36/1  "Age"
  raptor_can_rxmsg16/2 -> Bus Creator16/2  "BMS_counterMsg514"
  Bus Creator56/1 -> Bus Creator5/59  "IO_CAN2_558_Bus"
  raptor_can_rxmsg9/4 -> Bus Creator50/4  "BMS_module1Cell5Volt"
  raptor_can_rxmsg6/3 -> Bus Creator7/3  "BMS_module1Volt"
  Bus Creator23/1 -> Bus Creator5/26  "IO_CAN2_525_Bus"
  Bus Creator46/1 -> Bus Creator5/43  "IO_CAN2_542_Bus"
  raptor_can_rxmsg43/3 -> Bus Creator43/3  "BMS_module4Cell1Volt"
  raptor_can_rxmsg11/2 -> Bus Creator11/2  "BMS_counterMsg515"
  raptor_can_rxmsg33/1 -> Bus Creator33/1  "Age"
  raptor_can_rxmsg31/4 -> Bus Creator31/4  "BMS_module3Cell2Temp"
  raptor_can_rxmsg60/4 -> Bus Creator61/4  "BMS_module1Cell8Volt"
  raptor_can_rxmsg62/1 -> Bus Creator63/1  "Age"
  raptor_can_rxmsg13/1 -> Bus Creator13/1  "Age"
  raptor_can_rxmsg5/1 -> Bus Creator6/1  "Age"
  raptor_can_rxmsg45/5 -> Bus Creator45/5  "BMS_module4Cell9Volt"
  raptor_can_rxmsg50/5 -> Bus Creator51/5  "BMS_module3Cell9Volt"
  Bus Creator45/1 -> Bus Creator5/42  "IO_CAN2_541_Bus"
  raptor_can_rxmsg61/3 -> Bus Creator62/3  "BMS_module5Cell7Volt"
  raptor_can_rxmsg20/1 -> Bus Creator20/1  "Age"
  raptor_can_rxmsg62/3 -> Bus Creator63/3  "BMS_module5Cell10Volt"
  Bus Creator9/1 -> Bus Creator5/4  "IO_CAN1_503_Bus"
  raptor_can_rxmsg50/3 -> Bus Creator51/3  "BMS_module3Cell7Volt"
  raptor_can_rxmsg9/2 -> Bus Creator50/2  "BMS_counterMsg504"
  raptor_can_rxmsg37/5 -> Bus Creator37/5  "BMS_module4Cell15Temp"
  raptor_can_rxmsg28/5 -> Bus Creator28/5  "BMS_module5Cell15Volt"
  Bus Creator34/1 -> Bus Creator5/37  "IO_CAN2_536_Bus"
  raptor_can_rxmsg19/3 -> Bus Creator19/3  "BMS_module2Cell1Temp"
  raptor_can_rxmsg34/4 -> Bus Creator34/4  "BMS_module3Cell11Temp"
  raptor_can_rxmsg64/5 -> Bus Creator65/5  "BMS_module5Cell15Temp"
  Bus Creator62/1 -> Bus Creator5/54  "IO_CAN2_553_Bus"
  raptor_can_rxmsg65/4 -> Bus Creator66/4  "BMS_module1Cell11Volt"
  raptor_can_rxmsg65/3 -> Bus Creator66/3  "BMS_module1Cell10Volt"
  raptor_can_rxmsg49/4 -> Bus Creator49/4  "BMS_module3Cell5Volt"
  Bus Creator49/1 -> Bus Creator5/29  "IO_CAN2_528_Bus"
  raptor_can_rxmsg54/2 -> Bus Creator55/2  "BMS_counterMsg557"
  raptor_can_rxmsg52/1 -> Bus Creator53/1  "Age"
  raptor_can_rxmsg34/1 -> Bus Creator34/1  "Age"
  raptor_can_rxmsg12/2 -> Bus Creator12/2  "BMS_counterMsg510"
  raptor_can_rxmsg62/2 -> Bus Creator63/2  "BMS_counterMsg554"
  raptor_can_rxmsg49/3 -> Bus Creator49/3  "BMS_module3Cell4Volt"
  raptor_can_rxmsg40/2 -> Bus Creator40/2  "BMS_counterMsg546"
  raptor_can_rxmsg46/4 -> Bus Creator46/4  "BMS_module4Cell11Volt"
  raptor_can_rxmsg33/5 -> Bus Creator33/5  "BMS_module3Cell9Temp"
  raptor_can_rxmsg67/5 -> Bus Creator68/5  "BMS_module1Cell18Volt"
  raptor_can_rxmsg38/1 -> Bus Creator38/1  "Age"
  raptor_can_rxmsg65/1 -> Bus Creator66/1  "Age"
  raptor_can_rxmsg63/5 -> Bus Creator64/5  "BMS_module5Cell18Temp"
  Bus Creator21/1 -> Bus Creator5/24  "IO_CAN2_523_Bus"
  Bus Creator50/1 -> Bus Creator5/5  "IO_CAN2_504_Bus"
  raptor_can_rxmsg30/3 -> Bus Creator30/3  "BMS_module3Cell16Temp"
  raptor_can_rxmsg29/5 -> Bus Creator29/5  "BMS_module3Cell18Volt"
  raptor_can_rxmsg32/1 -> Bus Creator32/1  "Age"
  raptor_can_rxmsg54/4 -> Bus Creator55/4  "BMS_module5Cell2Temp"
  raptor_can_rxmsg7/3 -> Bus Creator8/3  "BMS_module4Volt"
  Bus Creator22/1 -> Bus Creator5/25  "IO_CAN2_524_Bus"
  raptor_can_rxmsg27/1 -> Bus Creator27/1  "Age"
  raptor_can_rxmsg45/3 -> Bus Creator45/3  "BMS_module4Cell7Volt"
  raptor_can_rxmsg21/5 -> Bus Creator21/5  "BMS_module2Cell9Temp"
  raptor_can_rxmsg50/4 -> Bus Creator51/4  "BMS_module3Cell8Volt"
  raptor_can_rxmsg17/4 -> Bus Creator17/4  "BMS_module2Cell17Volt"
  raptor_can_rxmsg7/2 -> Bus Creator8/2  "BMS_counterMsg502"
  raptor_can_rxmsg9/3 -> Bus Creator50/3  "BMS_module1Cell4Volt"
  raptor_can_rxmsg24/5 -> Bus Creator24/5  "BMS_module2Cell6Volt"
  raptor_can_rxmsg53/3 -> Bus Creator54/3  "BMS_module5Cell16Volt"
  raptor_can_rxmsg39/4 -> Bus Creator39/4  "BMS_module5Cell11Temp"
  raptor_can_rxmsg44/2 -> Bus Creator44/2  "BMS_counterMsg540"
  raptor_can_rxmsg21/4 -> Bus Creator21/4  "BMS_module2Cell8Temp"
  raptor_can_rxmsg65/5 -> Bus Creator66/5  "BMS_module1Cell12Volt"
  raptor_can_rxmsg29/2 -> Bus Creator29/2  "BMS_counterMsg532"
  raptor_can_rxmsg23/3 -> Bus Creator23/3  "BMS_module2Cell13Temp"
  raptor_can_rxmsg51/3 -> Bus Creator52/3  "BMS_module3Cell10Volt"
  raptor_can_rxmsg55/5 -> Bus Creator56/5  "BMS_module5Cell6Temp"
  raptor_can_rxmsg40/3 -> Bus Creator40/3  "BMS_module4Cell4Temp"
  raptor_can_rxmsg21/3 -> Bus Creator21/3  "BMS_module2Cell7Temp"
  raptor_can_rxmsg60/3 -> Bus Creator61/3  "BMS_module1Cell7Volt"
  raptor_can_rxmsg22/3 -> Bus Creator22/3  "BMS_module2Cell10Temp"
  raptor_can_rxmsg54/3 -> Bus Creator55/3  "BMS_module5Cell1Temp"
  raptor_can_rxmsg52/5 -> Bus Creator53/5  "BMS_module3Cell15Volt"
  raptor_can_rxmsg62/4 -> Bus Creator63/4  "BMS_module5Cell11Volt"
  raptor_can_rxmsg61/5 -> Bus Creator62/5  "BMS_module5Cell9Volt"
  raptor_can_rxmsg61/1 -> Bus Creator62/1  "Age"
  raptor_can_rxmsg46/5 -> Bus Creator46/5  "BMS_module4Cell12Volt"
  raptor_can_rxmsg20/5 -> Bus Creator20/5  "BMS_module2Cell6Temp"
  raptor_can_rxmsg47/1 -> Bus Creator47/1  "Age"
  Bus Creator38/1 -> Bus Creator5/46  "IO_CAN2_545_Bus"
  raptor_can_rxmsg67/3 -> Bus Creator68/3  "BMS_module1Cell16Volt"
  raptor_can_rxmsg65/2 -> Bus Creator66/2  "BMS_counterMsg506"
  raptor_can_rxmsg13/4 -> Bus Creator13/4  "BMS_module1Cell8Temp"
  raptor_can_rxmsg28/1 -> Bus Creator28/1  "Age"
  raptor_can_rxmsg58/5 -> Bus Creator59/5  "BMS_module5Cell3Volt"
  raptor_can_rxmsg37/4 -> Bus Creator37/4  "BMS_module4Cell14Temp"
  raptor_can_rxmsg53/1 -> Bus Creator54/1  "Age"
  raptor_can_rxmsg21/2 -> Bus Creator21/2  "BMS_counterMsg523"
  raptor_can_rxmsg28/2 -> Bus Creator28/2  "BMS_counterMsg555"
  raptor_can_rxmsg42/3 -> Bus Creator42/3  "BMS_module4Cell10Temp"
  raptor_can_rxmsg15/3 -> Bus Creator15/3  "BMS_module1Cell13Temp"
  raptor_can_rxmsg50/2 -> Bus Creator51/2  "BMS_counterMsg529"
  Bus Creator18/1 -> Bus Creator5/27  "IO_CAN2_526_Bus"
  raptor_can_rxmsg51/2 -> Bus Creator52/2  "BMS_counterMsg530"
  raptor_can_rxmsg49/1 -> Bus Creator49/1  "Age"
  raptor_can_rxmsg56/5 -> Bus Creator57/5  "BMS_module5Cell9Temp"
  raptor_can_rxmsg29/4 -> Bus Creator29/4  "BMS_module3Cell17Volt"
  raptor_can_rxmsg67/2 -> Bus Creator68/2  "BMS_counterMsg508"
  raptor_can_rxmsg42/2 -> Bus Creator42/2  "BMS_counterMsg548"
  raptor_can_rxmsg8/2 -> Bus Creator9/2  "BMS_counterMsg503"
  Bus Creator6/1 -> Bus Creator5/1  "IO_CAN2_500_Bus"
  raptor_can_rxmsg42/4 -> Bus Creator42/4  "BMS_module4Cell11Temp"
  raptor_can_rxmsg64/4 -> Bus Creator65/4  "BMS_module5Cell14Temp"
  raptor_can_rxmsg45/1 -> Bus Creator45/1  "Age"
  raptor_can_rxmsg60/2 -> Bus Creator61/2  "BMS_counterMsg505"
  raptor_can_rxmsg34/3 -> Bus Creator34/3  "BMS_module3Cell10Temp"
  raptor_can_rxmsg58/4 -> Bus Creator59/4  "BMS_module5Cell2Volt"
  raptor_can_rxmsg66/4 -> Bus Creator67/4  "BMS_module1Cell14Volt"
  raptor_can_rxmsg61/2 -> Bus Creator62/2  "BMS_counterMsg553"
  Bus Creator19/1 -> Bus Creator5/22  "IO_CAN2_521_Bus"
  raptor_can_rxmsg18/2 -> Bus Creator18/2  "BMS_counterMsg526"
  raptor_can_rxmsg46/3 -> Bus Creator46/3  "BMS_module4Cell10Volt"
  raptor_can_rxmsg5/4 -> Bus Creator6/4  "BMS_packCurr"
  raptor_can_rxmsg49/2 -> Bus Creator49/2  "BMS_counterMsg528"
  raptor_can_rxmsg12/4 -> Bus Creator12/4  "BMS_module1Cell5Temp"
  raptor_can_rxmsg17/3 -> Bus Creator17/3  "BMS_module2Cell16Volt"
  raptor_can_rxmsg31/5 -> Bus Creator31/5  "BMS_module3Cell3Temp"
  raptor_can_rxmsg39/1 -> Bus Creator39/1  "Age"
  raptor_can_rxmsg47/3 -> Bus Creator47/3  "BMS_module4Cell13Volt"
  raptor_can_rxmsg28/3 -> Bus Creator28/3  "BMS_module5Cell13Volt"
  raptor_can_rxmsg35/5 -> Bus Creator35/5  "BMS_module3Cell15Temp"
  raptor_can_rxmsg14/2 -> Bus Creator14/2  "BMS_counterMsg512"
  raptor_can_rxmsg25/5 -> Bus Creator25/5  "BMS_module2Cell9Volt"
  Bus Creator65/1 -> Bus Creator5/62  "IO_CAN2_561_Bus"
  raptor_can_rxmsg10/5 -> Bus Creator10/5  "BMS_module1Cell3Temp"
  raptor_can_rxmsg13/5 -> Bus Creator13/5  "BMS_module1Cell9Temp"
  raptor_can_rxmsg23/4 -> Bus Creator23/4  "BMS_module2Cell14Temp"
  raptor_can_rxmsg14/4 -> Bus Creator14/4  "BMS_module1Cell11Temp"
  raptor_can_rxmsg10/1 -> Bus Creator10/1  "Age"
  raptor_can_rxmsg53/4 -> Bus Creator54/4  "BMS_module5Cell17Volt"
  raptor_can_rxmsg60/1 -> Bus Creator61/1  "Age"
  raptor_can_rxmsg36/3 -> Bus Creator36/3  "BMS_module4Cell16Volt"
  raptor_can_rxmsg18/1 -> Bus Creator18/1  "Age"
  raptor_can_rxmsg32/3 -> Bus Creator32/3  "BMS_module3Cell4Temp"
  raptor_can_rxmsg34/5 -> Bus Creator34/5  "BMS_module3Cell12Temp"
  Bus Creator15/1 -> Bus Creator5/14  "IO_CAN2_513_Bus"
  raptor_can_rxmsg12/3 -> Bus Creator12/3  "BMS_module1Cell4Temp"
  raptor_can_rxmsg32/4 -> Bus Creator32/4  "BMS_module3Cell5Temp"
  raptor_can_rxmsg11/5 -> Bus Creator11/5  "BMS_module2Cell3Volt"
  raptor_can_rxmsg18/5 -> Bus Creator18/5  "BMS_module2Cell18Temp"
  raptor_can_rxmsg48/1 -> Bus Creator48/1  "Age"
  Bus Creator25/1 -> Bus Creator5/18  "IO_CAN2_517_Bus"
  raptor_can_rxmsg58/1 -> Bus Creator59/1  "Age"
  raptor_can_rxmsg32/2 -> Bus Creator32/2  "BMS_counterMsg534"
  Bus Creator61/1 -> Bus Creator5/6  "IO_CAN2_505_Bus"
  raptor_can_rxmsg30/1 -> Bus Creator30/1  "Age"
  raptor_can_rxmsg44/1 -> Bus Creator44/1  "Age"
  raptor_can_rxmsg25/2 -> Bus Creator25/2  "BMS_counterMsg517"
  raptor_can_rxmsg15/4 -> Bus Creator15/4  "BMS_module1Cell14Temp"
  Bus Creator52/1 -> Bus Creator5/31  "IO_CAN2_530_Bus"
  Bus Creator11/1 -> Bus Creator5/16  "IO_CAN2_515_Bus"
  raptor_can_rxmsg66/3 -> Bus Creator67/3  "BMS_module1Cell13Volt"
  Bus Creator27/1 -> Bus Creator5/20  "IO_CAN2_519_Bus"
  raptor_can_rxmsg26/1 -> Bus Creator26/1  "Age"
  raptor_can_rxmsg56/2 -> Bus Creator57/2  "BMS_counterMsg559"
  raptor_can_rxmsg8/4 -> Bus Creator9/4  "BMS_module1Cell2Volt"
  raptor_can_rxmsg39/3 -> Bus Creator39/3  "BMS_module5Cell10Temp"
  raptor_can_rxmsg35/4 -> Bus Creator35/4  "BMS_module3Cell14Temp"
  raptor_can_rxmsg31/2 -> Bus Creator31/2  "BMS_counterMsg533"
  raptor_can_rxmsg50/1 -> Bus Creator51/1  "Age"
  raptor_can_rxmsg67/4 -> Bus Creator68/4  "BMS_module1Cell17Volt"
  raptor_can_rxmsg26/3 -> Bus Creator26/3  "BMS_module2Cell10Volt"
  raptor_can_rxmsg25/1 -> Bus Creator25/1  "Age"
  raptor_can_rxmsg8/1 -> Bus Creator9/1  "Age"
  raptor_can_rxmsg11/4 -> Bus Creator11/4  "BMS_module2Cell2Volt"
  raptor_can_rxmsg41/4 -> Bus Creator41/4  "BMS_module4Cell8Temp"
  Bus Creator67/1 -> Bus Creator5/8  "IO_CAN2_507_Bus"
  raptor_can_rxmsg22/5 -> Bus Creator22/5  "BMS_module2Cell12Temp"
  raptor_can_rxmsg51/4 -> Bus Creator52/4  "BMS_module3Cell11Volt"
  raptor_can_rxmsg46/2 -> Bus Creator46/2  "BMS_counterMsg542"
  raptor_can_rxmsg18/3 -> Bus Creator18/3  "BMS_module2Cell16Temp"
  raptor_can_rxmsg7/1 -> Bus Creator8/1  "Age"
  raptor_can_rxmsg12/1 -> Bus Creator12/1  "Age"
  raptor_can_rxmsg54/5 -> Bus Creator55/5  "BMS_module5Cell3Temp"
  raptor_can_rxmsg37/2 -> Bus Creator37/2  "BMS_counterMsg549"
  raptor_can_rxmsg37/3 -> Bus Creator37/3  "BMS_module4Cell13Temp"
  Bus Creator43/1 -> Bus Creator5/40  "IO_CAN2_539_Bus"
  raptor_can_rxmsg66/2 -> Bus Creator67/2  "BMS_counterMsg507"
  raptor_can_rxmsg20/3 -> Bus Creator20/3  "BMS_module2Cell4Temp"
  raptor_can_rxmsg36/2 -> Bus Creator36/2  "BMS_counterMsg544"
  raptor_can_rxmsg12/5 -> Bus Creator12/5  "BMS_module1Cell6Temp"
  Bus Creator35/1 -> Bus Creator5/38  "IO_CAN2_537_Bus"
  raptor_can_rxmsg61/4 -> Bus Creator62/4  "BMS_module5Cell8Volt"
  raptor_can_rxmsg11/3 -> Bus Creator11/3  "BMS_module2Cell1Volt"
  raptor_can_rxmsg27/4 -> Bus Creator27/4  "BMS_module2Cell14Volt"
  Bus Creator32/1 -> Bus Creator5/35  "IO_CAN2_534_Bus"
  raptor_can_rxmsg27/2 -> Bus Creator27/2  "BMS_counterMsg519"
  raptor_can_rxmsg25/4 -> Bus Creator25/4  "BMS_module2Cell8Volt"
  raptor_can_rxmsg44/4 -> Bus Creator44/4  "BMS_module4Cell5Volt"
  raptor_can_rxmsg44/3 -> Bus Creator44/3  "BMS_module4Cell4Volt"
  raptor_can_rxmsg52/4 -> Bus Creator53/4  "BMS_module3Cell14Volt"
  Bus Creator20/1 -> Bus Creator5/23  "IO_CAN2_522_Bus"
  raptor_can_rxmsg63/1 -> Bus Creator64/1  "Age"
  raptor_can_rxmsg26/2 -> Bus Creator26/2  "BMS_counterMsg518"
  Bus Creator33/1 -> Bus Creator5/36  "IO_CAN2_535_Bus"
  raptor_can_rxmsg52/3 -> Bus Creator53/3  "BMS_module3Cell13Volt"
  Bus Creator26/1 -> Bus Creator5/19  "IO_CAN2_518_Bus"
  raptor_can_rxmsg23/2 -> Bus Creator23/2  "BMS_counterMsg525"
  raptor_can_rxmsg38/4 -> Bus Creator38/4  "BMS_module4Cell2Temp"
  raptor_can_rxmsg55/3 -> Bus Creator56/3  "BMS_module5Cell4Temp"
  Bus Creator60/1 -> Bus Creator5/53  "IO_CAN2_552_Bus"
  raptor_can_rxmsg8/5 -> Bus Creator9/5  "BMS_module1Cell3Volt"
  Bus Creator12/1 -> Bus Creator5/11  "IO_CAN2_510_Bus"
  raptor_can_rxmsg41/5 -> Bus Creator41/5  "BMS_module4Cell9Temp"
  raptor_can_rxmsg48/5 -> Bus Creator48/5  "BMS_module3Cell3Volt"
  raptor_can_rxmsg16/3 -> Bus Creator16/3  "BMS_module1Cell16Temp"
  raptor_can_rxmsg38/2 -> Bus Creator38/2  "BMS_counterMsg545"
  Bus Creator8/1 -> Bus Creator5/3  "IO_CAN2_502_Bus"
  raptor_can_rxmsg66/5 -> Bus Creator67/5  "BMS_module1Cell15Volt"
  raptor_can_rxmsg9/1 -> Bus Creator50/1  "Age"
  Bus Creator29/1 -> Bus Creator5/33  "IO_CAN2_532_Bus"
  raptor_can_rxmsg30/5 -> Bus Creator30/5  "BMS_module3Cell18Temp"
  raptor_can_rxmsg36/4 -> Bus Creator36/4  "BMS_module4Cell17Volt"
  Bus Creator31/1 -> Bus Creator5/34  "IO_CAN2_533_Bus"
  raptor_can_rxmsg30/4 -> Bus Creator30/4  "BMS_module3Cell17Temp"
  raptor_can_rxmsg45/2 -> Bus Creator45/2  "BMS_counterMsg541"
  Bus Creator16/1 -> Bus Creator5/15  "IO_CAN2_514_Bus"
  raptor_can_rxmsg59/1 -> Bus Creator60/1  "Age"
  raptor_can_rxmsg6/1 -> Bus Creator7/1  "Age"
  Bus Creator53/1 -> Bus Creator5/32  "IO_CAN2_531_Bus"
  raptor_can_rxmsg9/5 -> Bus Creator50/5  "BMS_module1Cell6Volt"
  raptor_can_rxmsg47/2 -> Bus Creator47/2  "BMS_counterMsg543"
  raptor_can_rxmsg41/3 -> Bus Creator41/3  "BMS_module4Cell7Temp"
  raptor_can_rxmsg13/2 -> Bus Creator13/2  "BMS_counterMsg511"
  raptor_can_rxmsg56/3 -> Bus Creator57/3  "BMS_module5Cell7Temp"
  raptor_can_rxmsg31/3 -> Bus Creator31/3  "BMS_module3Cell1Temp"
  raptor_can_rxmsg57/1 -> Bus Creator58/1  "Age"
  raptor_can_rxmsg55/2 -> Bus Creator56/2  "BMS_counterMsg558"
  raptor_can_rxmsg5/2 -> Bus Creator6/2  "BMS_counterMsg500"
  raptor_can_rxmsg15/5 -> Bus Creator15/5  "BMS_module1Cell15Temp"
  raptor_can_rxmsg17/2 -> Bus Creator17/2  "BMS_counterMsg520"
  raptor_can_rxmsg53/5 -> Bus Creator54/5  "BMS_module5Cell18Volt"
  Bus Creator59/1 -> Bus Creator5/52  "IO_CAN2_551_Bus"
  raptor_can_rxmsg22/4 -> Bus Creator22/4  "BMS_module2Cell11Temp"
  raptor_can_rxmsg5/3 -> Bus Creator6/3  "BMS_packVoltage"
  raptor_can_rxmsg43/1 -> Bus Creator43/1  "Age"
  raptor_can_rxmsg32/5 -> Bus Creator32/5  "BMS_module3Cell6Temp"
  raptor_can_rxmsg15/2 -> Bus Creator15/2  "BMS_counterMsg513"
  raptor_can_rxmsg40/4 -> Bus Creator40/4  "BMS_module4Cell5Temp"
  raptor_can_rxmsg39/2 -> Bus Creator39/2  "BMS_counterMsg560"
  Bus Creator7/1 -> Bus Creator5/2  "IO_CAN2_501_Bus"
  raptor_can_rxmsg45/4 -> Bus Creator45/4  "BMS_module4Cell8Volt"
  raptor_can_rxmsg24/3 -> Bus Creator24/3  "BMS_module2Cell4Volt"
  raptor_can_rxmsg36/5 -> Bus Creator36/5  "BMS_module4Cell18Volt"
  raptor_can_rxmsg42/5 -> Bus Creator42/5  "BMS_module4Cell12Temp"
  raptor_can_rxmsg58/2 -> Bus Creator59/2  "BMS_counterMsg551"
  raptor_can_rxmsg20/4 -> Bus Creator20/4  "BMS_module2Cell5Temp"
  raptor_can_rxmsg13/3 -> Bus Creator13/3  "BMS_module1Cell7Temp"
  raptor_can_rxmsg33/4 -> Bus Creator33/4  "BMS_module3Cell8Temp"
  raptor_can_rxmsg56/4 -> Bus Creator57/4  "BMS_module5Cell8Temp"
  raptor_can_rxmsg10/3 -> Bus Creator10/3  "BMS_module1Cell1Temp"
  raptor_can_rxmsg19/5 -> Bus Creator19/5  "BMS_module2Cell3Temp"
  raptor_can_rxmsg31/1 -> Bus Creator31/1  "Age"
  raptor_can_rxmsg54/1 -> Bus Creator55/1  "Age"
  raptor_can_rxmsg41/1 -> Bus Creator41/1  "Age"
  raptor_can_rxmsg22/2 -> Bus Creator22/2  "BMS_counterMsg524"
  raptor_can_rxmsg57/3 -> Bus Creator58/3  "BMS_module4Cell16Temp"
  raptor_can_rxmsg29/3 -> Bus Creator29/3  "BMS_module3Cell16Volt"
  raptor_can_rxmsg34/2 -> Bus Creator34/2  "BMS_counterMsg536"
  raptor_can_rxmsg47/5 -> Bus Creator47/5  "BMS_module4Cell15Volt"
  raptor_can_rxmsg51/1 -> Bus Creator52/1  "Age"
  raptor_can_rxmsg19/1 -> Bus Creator19/1  "Age"
  raptor_can_rxmsg21/1 -> Bus Creator21/1  "Age"
  raptor_can_rxmsg41/2 -> Bus Creator41/2  "BMS_counterMsg547"
  Bus Creator41/1 -> Bus Creator5/48  "IO_CAN2_547_Bus"
  Bus Creator57/1 -> Bus Creator5/60  "IO_CAN2_559_Bus"
  Bus Creator54/1 -> Bus Creator5/57  "IO_CAN2_556_Bus"
  Bus Creator58/1 -> Bus Creator5/51  "IO_CAN2_550_Bus"
  Bus Creator55/1 -> Bus Creator5/58  "IO_CAN2_557_Bus"
  Bus Creator30/1 -> Bus Creator5/39  "IO_CAN2_538_Bus"
  Bus Creator42/1 -> Bus Creator5/49  "IO_CAN1_548_Bus"
  Bus Creator40/1 -> Bus Creator5/47  "IO_CAN2_546_Bus"
  Bus Creator28/1 -> Bus Creator5/56  "IO_CAN2_555_Bus"
  Bus Creator64/1 -> Bus Creator5/63  "IO_CAN2_562_Bus"
  Bus Creator63/1 -> Bus Creator5/55  "IO_CAN2_554_Bus"
